simulink model "LectureVersion_Stage02_Thermostat"  (R2021b)
settings: Solver=VariableStepAuto  StartTime=0.0  StopTime=10.0  RelTol=1e-3
model workspace (MAT data in the model file):
  M_heater_air = 3600
  T_heater = 50
  c_air = 1005.4
settings Model: Creator=jim  LastModifiedBy=jim

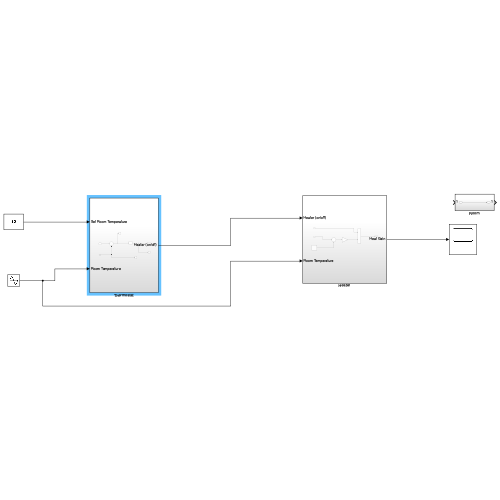
[thumbnail: Simulink's stored preview of the top-level diagram]
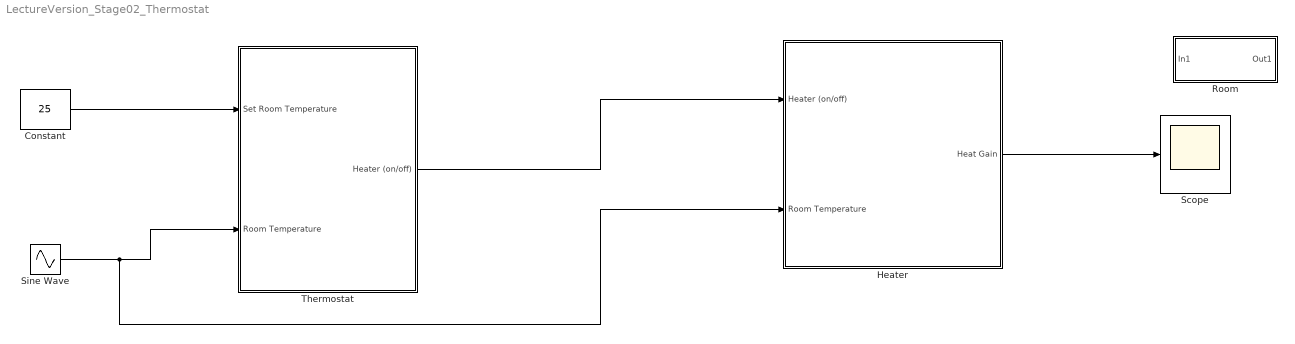
== system LectureVersion_Stage02_Thermostat ==
  Constant : Constant  Value=25
  Heater : Subsystem
  Room : Subsystem
  Scope : Scope
  Sine Wave : Sin  Amplitude=10  Bias=20  Frequency=0.5  SampleTime=0
  Thermostat : Subsystem
  wires:
  Heater/1(Heat Gain) -> Scope/1
  Constant/1 -> Thermostat/1(Set Room Temperature)
  Sine Wave/1 -> Heater/2(Room Temperature), Thermostat/2(Room Temperature)
  Thermostat/1(Heater (on/off)) -> Heater/1(Heater (on/off))

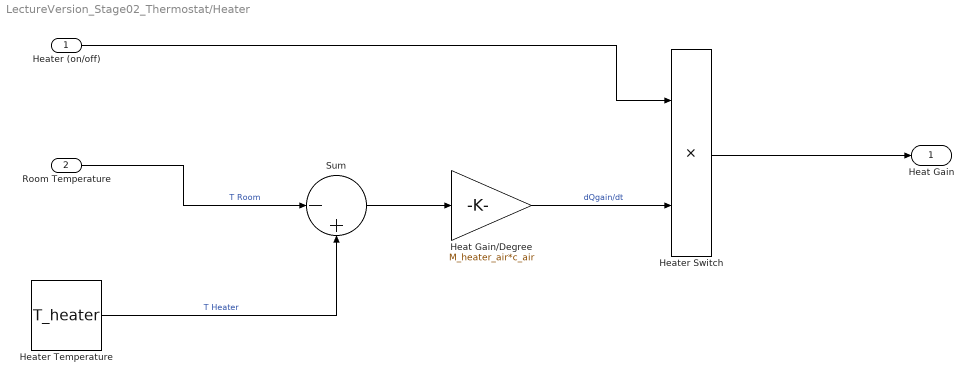
== system LectureVersion_Stage02_Thermostat/Heater ==
  Heater (on/off) : Inport
  Room Temperature : Inport  Port=2
  Heat Gain/Degree : Gain  Gain=M_heater_air*c_air
  Heater Switch : Product
  Heater Temperature : Constant  Value=T_heater
  Sum : Sum  Inputs=|-+
  Heat Gain : Outport
  wires:
  Sum/1 -> Heat Gain/Degree/1
  Room Temperature/1 -> Sum/1  "T Room"
  Heater Temperature/1 -> Sum/2  "T Heater"
  Heater (on/off)/1 -> Heater Switch/1
  Heater Switch/1 -> Heat Gain/1
  Heat Gain/Degree/1 -> Heater Switch/2  "dQgain/dt"

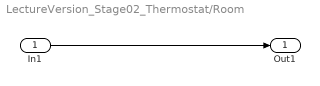
== system LectureVersion_Stage02_Thermostat/Room ==
  In1 : Inport
  Out1 : Outport
  wires:
  In1/1 -> Out1/1

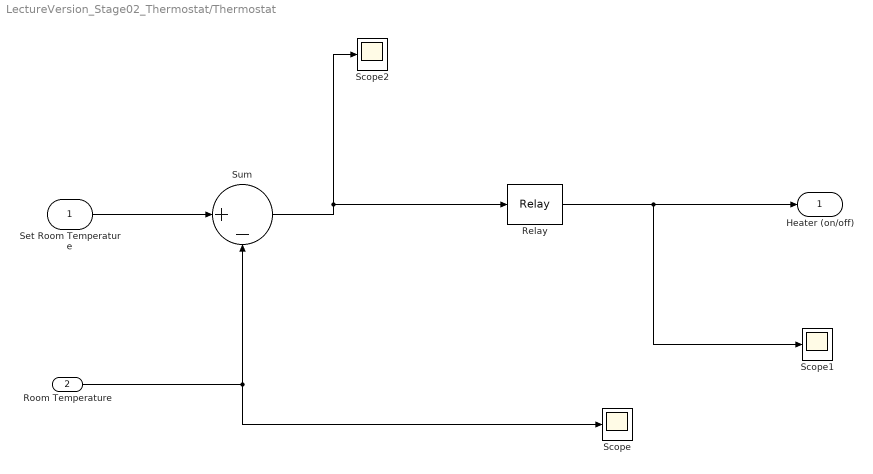
== system LectureVersion_Stage02_Thermostat/Thermostat ==
  Set Room Temperature : Inport
  Room Temperature : Inport  Port=2
  Relay : Relay  OnSwitchValue=2  OffSwitchValue=-2
  Scope : Scope
  Scope1 : Scope
  Scope2 : Scope
  Sum : Sum  Inputs=|+-
  Heater (on/off) : Outport
  wires:
  Set Room Temperature/1 -> Sum/1
  Room Temperature/1 -> Sum/2, Scope/1
  Sum/1 -> Relay/1, Scope2/1
  Relay/1 -> Scope1/1, Heater (on/off)/1
